simulink model "RPL_FLYSON"  (R2020b)
settings: Solver=VariableStepAuto  StartTime=0.0  StopTime=5.0  RelTol=1e-3
model workspace (MAT data in the model file):
  COM_DISTANCE_FROM_BOTTOM = 0.676
  CROSS_AREA = 0.25
  CURR_TEMP = 293
  DRAG_COEFF = 0.75
  MASS = 7
  P_SEA_LEVEL = 101325
  ROCKET_HEIGHT = 1.352
  R_AIR = 287.058
libraries: vrlib x2, shared6dof x1, simulink x1, sharedutil x1, sharedtransform x1
settings Model: OrderedModelArguments=off  Creator=Adam  LastModifiedBy=Adam

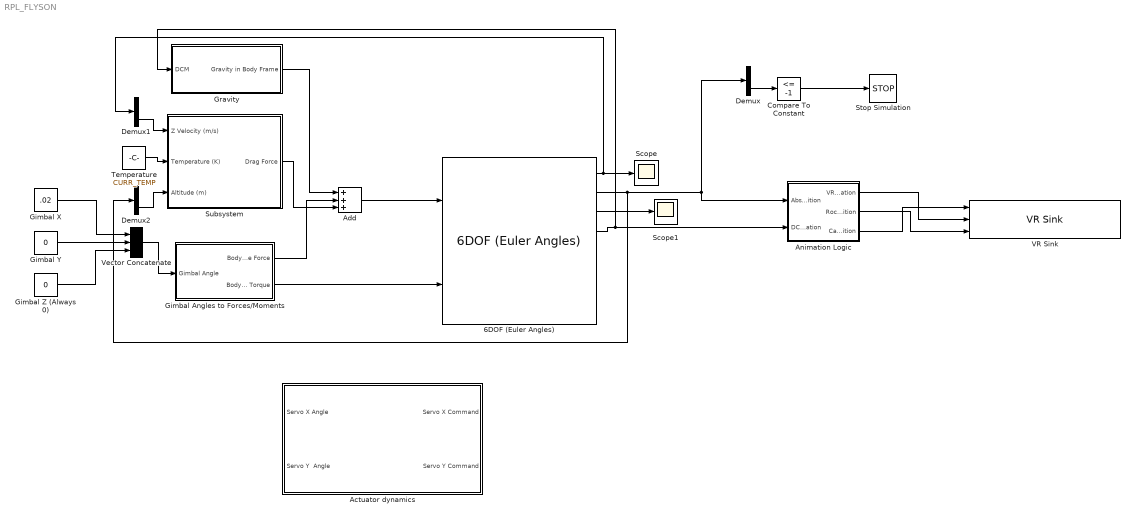
== system RPL_FLYSON ==
  6DOF (Euler Angles) : shared6dof/6DOF (Euler Angles)  units=Metric (MKS)  mtype=Fixed  rep=Euler Angles  xme_0=[0 0 0]  Vm_0=[0 0 0]  eul_0=[0 0 0]  pm_0=[0 0 0]  mass_0=MASS  mass_e=0.5  mass_f=2.0  inertia=eye(3)  inertia_e=eye(3)  inertia_f=2*eye(3)  k_quat=1.0  vre_flag=on  abi_flag=off  aMode=0  xme_statename=''  Vm_statename=''  eul_statename=''  quat_statename=''  pm_statename=''  mass_statename=''
      settings: SourceProductBaseCode=AE,PW,MT,UV,VE,VP
  Actuator dynamics : Subsystem
  Add : Sum  Inputs=+++
  Animation Logic : Subsystem
  Compare To Constant : simulink/Logic and Bit Operations/Compare To Constant  relop=<=  const=-1  OutDataTypeStr=boolean
  Demux : Demux  Outputs=3
  Demux1 : Demux  Outputs=3
  Demux2 : Demux  Outputs=3
  Gimbal Angles to Forces/Moments : Subsystem
  Gimbal X : Constant  Value=.02
  Gimbal Y : Constant  Value=0
  Gimbal Z (Always 0) : Constant  Value=0
  Gravity : Subsystem
  Scope : Scope
  Scope1 : Scope
  Stop Simulation : Stop
  Subsystem : Subsystem
  Temperature : Constant  Value=CURR_TEMP
  VR Sink : vrlib/VR Sink  InstantiateOnLoad=on  SampleTime=0.001  ViewEnable=on  RemoteChange=off  RemoteView=off  FieldsWritten=Camera.position.3.1.1.double#Exported_Transform.rotation.4.1.1.double#Exported_Transform.translation.3.1.1.double  WorldFileName=FLYSON_3D.wrl  AutoView=on  VideoDimensions=[]  AllowVariableSize=off  FigureProperties="{'Position', 'Name', 'Viewpoint', 'CameraBound', 'CameraDirection', 'CameraPosition', 'CameraUpVector', 'ZoomFactor', 'Antialiasing', 'Headlight', 'Lighting', 'NavPanel', 'Sound', 'StatusBar', 'Stereo3D', 'Stereo3DCameraOffset', 'Stereo3DHIT', 'ToolBar', 'Textures', 'Transparency', 'Triad', 'Wireframe', 'NavZones', 'NavMode', 'NavSpeed', 'CaptureFileFormat', 'CaptureFileName', 'Record2DCompressMethod', 'Record2DCompressQuality', 'Record2D', 'Record2DFileName', 'Record2DFPS'; [5.0000000000000000e+00   9.2000000000000000e+01   5.7600000000000000e+02   3.5000000000000000e+02], '', '_untitled_1', 'on', [0.0000000000000000e+00   0.0000000000000000e+00  -1.0000000000000000e+00], [0.0000000000000000e+00   0.0000000000000000e+00   0.0000000000000000e+00], [0.0000000000000000e+00   1.0000000000000000e+00   0.0000000000000000e+00], [1.0000000000000000e+00], 'on', 'on', 'on', 'halfbar', 'on', 'on', 'off', [1.0000000149011612e-01], [0.0000000000000000e+00], 'on', 'on', 'on', 'none', 'off', 'off', 'fly', 'normal', 'tif', '%f_anim_%n.tif', 'auto', [7.5000000000000000e+01], 'off', '%f_anim_%n.avi', 'auto'}"
  Vector Concatenate : Concatenate  NumInputs=3
  wires:
  Add/1 -> 6DOF (Euler Angles)/1
  6DOF (Euler Angles)/1 -> Demux1/1, Scope/1
  Gimbal Angles to Forces/Moments/1(Body-Frame Force) -> Add/2
  Gimbal Angles to Forces/Moments/2(Body-Frame Torque) -> 6DOF (Euler Angles)/2
  6DOF (Euler Angles)/3 -> Scope1/1
  6DOF (Euler Angles)/2 -> Demux2/1, Demux/1, Animation Logic/1(Absolute Position)
  6DOF (Euler Angles)/4 -> Gravity/1(DCM), Animation Logic/2(DCM Rotation)
  Gravity/1(Gravity in Body Frame) -> Add/1
  Animation Logic/3(Camera Position) -> VR Sink/1
  Animation Logic/1(VR Rotation) -> VR Sink/2
  Animation Logic/2(Rocket Position) -> VR Sink/3
  Gimbal Z (Always 0)/1 -> Vector Concatenate/3
  Vector Concatenate/1 -> Gimbal Angles to Forces/Moments/1(Gimbal Angle)
  Gimbal X/1 -> Vector Concatenate/1
  Gimbal Y/1 -> Vector Concatenate/2
  Demux/3 -> Compare To Constant/1
  Compare To Constant/1 -> Stop Simulation/1
  Subsystem/1(Drag Force) -> Add/3
  Temperature/1 -> Subsystem/2(Temperature (K))
  Demux1/3 -> Subsystem/1(Z Velocity (m/s))
  Demux2/3 -> Subsystem/3(Altitude (m))

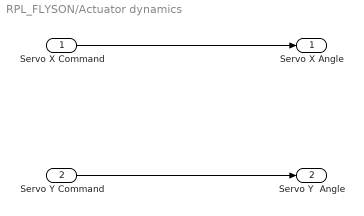
== system RPL_FLYSON/Actuator dynamics ==
  Servo X Command : Inport
  Servo Y Command : Inport  Port=2
  Servo X Angle : Outport
  Servo Y  Angle : Outport  Port=2
  wires:
  Servo X Command/1 -> Servo X Angle/1
  Servo Y Command/1 -> Servo Y  Angle/1

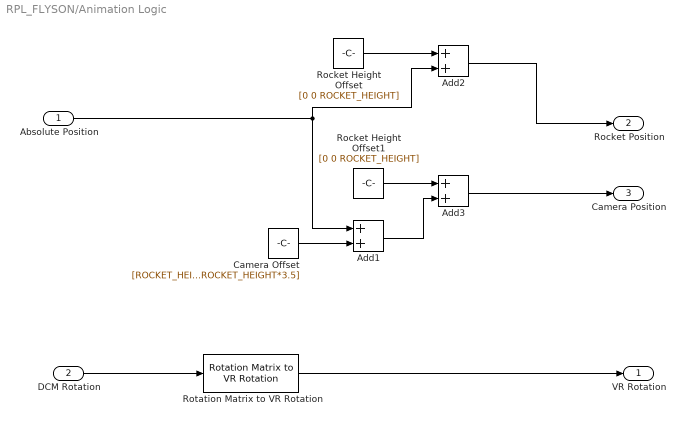
== system RPL_FLYSON/Animation Logic ==
  Absolute Position : Inport
  DCM Rotation : Inport  Port=2
  Add1 : Sum
  Add2 : Sum
  Add3 : Sum
  Camera Offset : Constant  Value=[ROCKET_HEIGHT*5 0 ROCKET_HEIGHT*3.5]
  Rocket Height Offset : Constant  Value=[0 0 ROCKET_HEIGHT]
  Rocket Height Offset1 : Constant  Value=[0 0 ROCKET_HEIGHT]
  Rotation Matrix to VR Rotation : vrlib/Utilities/Rotation Matrix to VR Rotation  maxzero=1e-12
      settings: SourceProductBaseCode=SL
  VR Rotation : Outport
  Rocket Position : Outport  Port=2
  Camera Position : Outport  Port=3
  wires:
  Add2/1 -> Rocket Position/1
  Add3/1 -> Camera Position/1
  Rocket Height Offset1/1 -> Add3/1
  Camera Offset/1 -> Add1/2
  DCM Rotation/1 -> Rotation Matrix to VR Rotation/1
  Add1/1 -> Add3/2
  Absolute Position/1 -> Add2/2, Add1/1
  Rocket Height Offset/1 -> Add2/1
  Rotation Matrix to VR Rotation/1 -> VR Rotation/1

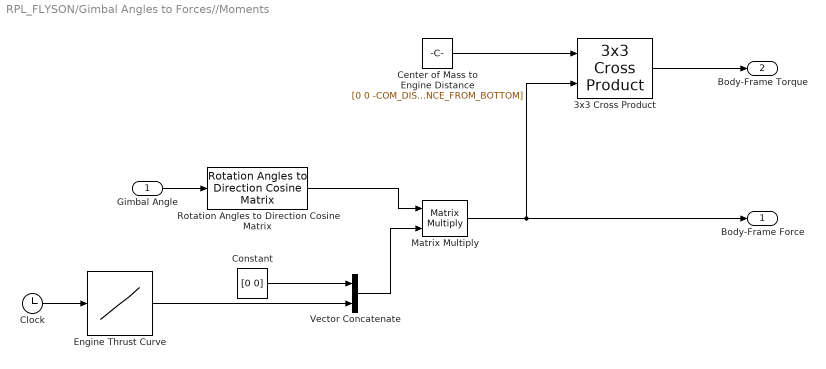
== system RPL_FLYSON/Gimbal Angles to Forces//Moments ==
  Gimbal Angle : Inport
  3x3 Cross Product : sharedutil/3x3 Cross Product  aMode=aMode
      settings: SourceProductBaseCode=AE,PW,MT,UV,VE,VP
  Center of Mass to Engine Distance : Constant  Value=[0 0 -COM_DISTANCE_FROM_BOTTOM]
  Clock : Clock
  Constant : Constant  Value=[0 0]
  Engine Thrust Curve : Lookup_n-D  NumberOfTableDimensions=1  BreakpointsForDimension1=[0:8] / 2  Table=[200 400 400 300 50 20 10 0 0]  InterpMethod=Linear Lagrange  InternalRulePriority=Speed  RndMeth=Simplest  InputSameDT=on
  Matrix Multiply : Product  Multiplication=Matrix(*)
  Rotation Angles to Direction Cosine Matrix : sharedtransform/Rotation Angles to Direction Cosine Matrix  rotationOrder=XYZ  aMode=aMode
      settings: SourceProductBaseCode=AE,PW,MT,UV,VE,VP
  Vector Concatenate : Concatenate
  Body-Frame Force : Outport
  Body-Frame Torque : Outport  Port=2
  wires:
  Gimbal Angle/1 -> Rotation Angles to Direction Cosine Matrix/1
  Center of Mass to Engine Distance/1 -> 3x3 Cross Product/1
  3x3 Cross Product/1 -> Body-Frame Torque/1
  Rotation Angles to Direction Cosine Matrix/1 -> Matrix Multiply/1
  Matrix Multiply/1 -> 3x3 Cross Product/2, Body-Frame Force/1
  Clock/1 -> Engine Thrust Curve/1
  Constant/1 -> Vector Concatenate/1
  Vector Concatenate/1 -> Matrix Multiply/2
  Engine Thrust Curve/1 -> Vector Concatenate/2

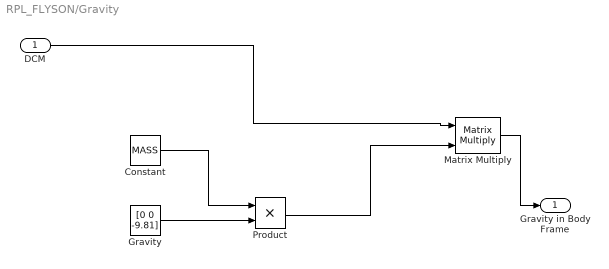
== system RPL_FLYSON/Gravity ==
  DCM : Inport
  Constant : Constant  Value=MASS
  Gravity : Constant  Value=[0 0 -9.81]
  Matrix Multiply : Product  Multiplication=Matrix(*)
  Product : Product
  Gravity in Body Frame : Outport
  wires:
  Gravity/1 -> Product/2
  Constant/1 -> Product/1
  Product/1 -> Matrix Multiply/2
  DCM/1 -> Matrix Multiply/1
  Matrix Multiply/1 -> Gravity in Body Frame/1

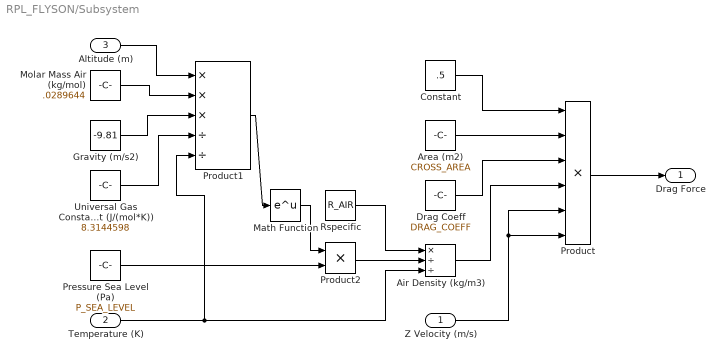
== system RPL_FLYSON/Subsystem ==
  Z Velocity (m/s) : Inport
  Temperature (K) : Inport  Port=2
  Altitude (m) : Inport  Port=3
  Air Density (kg/m3) : Product  Inputs=*//
  Area (m2) : Constant  Value=CROSS_AREA
  Constant : Constant  Value=.5
  Drag Coeff : Constant  Value=DRAG_COEFF
  Gravity (m/s2) : Constant  Value=-9.81
  Math Function : Math  SaturateOnIntegerOverflow=on
  Molar Mass Air (kg/mol) : Constant  Value=.0289644
  Pressure Sea Level (Pa) : Constant  Value=P_SEA_LEVEL
  Product : Product  Inputs=6
  Product1 : Product  Inputs=***//
  Product2 : Product
  Rspecific : Constant  Value=R_AIR
  Universal Gas Constant (J/(mol*K)) : Constant  Value=8.3144598
  Drag Force : Outport
  wires:
  Temperature (K)/1 -> Product1/5, Air Density (kg/m3)/3
  Rspecific/1 -> Air Density (kg/m3)/1
  Air Density (kg/m3)/1 -> Product/4
  Drag Coeff/1 -> Product/3
  Area (m2)/1 -> Product/2
  Constant/1 -> Product/1
  Z Velocity (m/s)/1 -> Product/6, Product/5
  Product/1 -> Drag Force/1
  Product2/1 -> Air Density (kg/m3)/2
  Math Function/1 -> Product2/1
  Gravity (m/s2)/1 -> Product1/3
  Molar Mass Air (kg/mol)/1 -> Product1/2
  Altitude (m)/1 -> Product1/1
  Universal Gas Constant (J/(mol*K))/1 -> Product1/4
  Product1/1 -> Math Function/1
  Pressure Sea Level (Pa)/1 -> Product2/2
